simulink library "INT_DrvDem_SetPoint"  (R2016b)
settings: Solver=VariableStepAuto  StartTime=0.0  StopTime=10.0  RelTol=1e-3
settings Model: Creator=xuxingpei  LastModifiedBy=xuxingpei

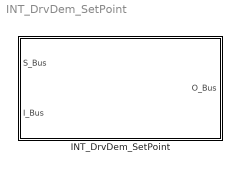
== system INT_DrvDem_SetPoint ==
  INT_DrvDem_SetPoint : Subsystem

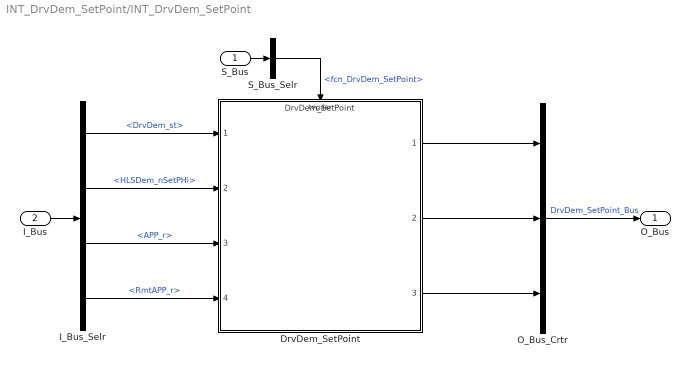
== system INT_DrvDem_SetPoint/INT_DrvDem_SetPoint ==
  S_Bus : Inport
  I_Bus : Inport  Port=2
  DrvDem_SetPoint : ModelReference  ModelNameDialog=DrvDem_SetPoint  SimulationMode=Normal  ModelReferenceVersion=1.79  TriggerPortName=function  TriggerPortTriggerType=function-call  TriggerPortStatesWhenEnabling=held
  I_Bus_Selr : BusSelector  OutputSignals=DrvDem_st,HLSDem_nSetPHi,APP_r,RmtAPP_r
  O_Bus_Crtr : BusCreator  Inputs=3
  S_Bus_Selr : BusSelector  OutputSignals=fcn_DrvDem_SetPoint
  O_Bus : Outport
  wires:
  S_Bus_Selr/1 -> DrvDem_SetPoint/Trigger  "<fcn_DrvDem_SetPoint>"
  S_Bus/1 -> S_Bus_Selr/1
  I_Bus/1 -> I_Bus_Selr/1
  I_Bus_Selr/1 -> DrvDem_SetPoint/1  "<DrvDem_st>"
  I_Bus_Selr/2 -> DrvDem_SetPoint/2  "<HLSDem_nSetPHi>"
  I_Bus_Selr/3 -> DrvDem_SetPoint/3  "<APP_r>"
  I_Bus_Selr/4 -> DrvDem_SetPoint/4  "<RmtAPP_r>"
  O_Bus_Crtr/1 -> O_Bus/1  "DrvDem_SetPoint_Bus"
  DrvDem_SetPoint/1 -> O_Bus_Crtr/1
  DrvDem_SetPoint/2 -> O_Bus_Crtr/2
  DrvDem_SetPoint/3 -> O_Bus_Crtr/3
